simulink model "model_p2"  (R2020b)
settings: Solver=VariableStepAuto  StartTime=0.0  StopTime=10  RelTol=1e-3
model workspace (MAT data in the model file):
  K1 = Simulink.Parameter
  K1.Value = 80000
  K1.DataType = 'auto'
  K1.Dimensions = [1 1]
  K2 = Simulink.Parameter
  K2.Value = 500000
  K2.DataType = 'auto'
  K2.Dimensions = [1 1]
  M1 = Simulink.Parameter
  M1.Value = 2500
  M1.DataType = 'auto'
  M1.Dimensions = [1 1]
  M2 = Simulink.Parameter
  M2.Value = 320
  M2.DataType = 'auto'
  M2.Dimensions = [1 1]
  b = Simulink.Parameter
  b.Value = 350
  b.DataType = 'auto'
  b.Dimensions = [1 1]
settings Model: OrderedModelArguments=off  Creator=ADMIN  LastModifiedBy=ADMIN
settings DataIOCC: ExternalInput=[t, stin]  LoadExternalInput=on  SaveFormat=Array

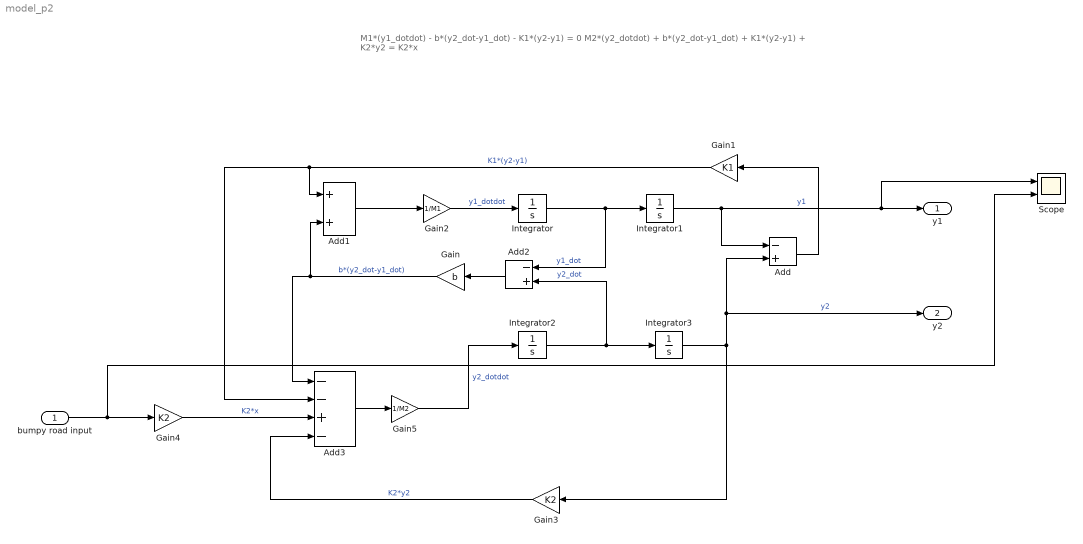
== system model_p2 ==
  note: M1*(y1_dotdot) - b*(y2_dot-y1_dot) - K1*(y2-y1) = 0
      |
      | M2*(y2_dotdot) + b*(y2_dot-y1_dot) + K1*(y2-y1) + K2*y2 = K2*x
  bumpy road input : Inport
  Add : Sum  Inputs=-+
  Add1 : Sum
  Add2 : Sum  Inputs=-+
  Add3 : Sum  Inputs=--+-
  Gain : Gain  Gain=b
  Gain1 : Gain  Gain=K1
  Gain2 : Gain  Gain=1/M1
  Gain3 : Gain  Gain=K2
  Gain4 : Gain  Gain=K2
  Gain5 : Gain  Gain=1/M2
  Integrator{,1..3} (4 alike) : Integrator
  Scope : Scope  NumInputPorts=2
  "y1 " : Outport
  y2 : Outport  Port=2
  wires:
  Gain2/1 -> Integrator/1  "y1_dotdot"
  Integrator/1 -> Add2/1, Integrator1/1  "y1_dot"
  Integrator1/1 -> Add/1, Scope/1, "y1 "/1  "y1"
  Integrator2/1 -> Add2/2, Integrator3/1  "y2_dot"
  Gain5/1 -> Integrator2/1  "y2_dotdot"
  Integrator3/1 -> Gain3/1, Add/2, y2/1  "y2"
  Add/1 -> Gain1/1
  Gain1/1 -> Add3/2, Add1/1  "K1*(y2-y1)"
  Add2/1 -> Gain/1
  Gain/1 -> Add3/1, Add1/2  "b*(y2_dot-y1_dot)"
  Add1/1 -> Gain2/1
  Gain3/1 -> Add3/4  "K2*y2"
  Add3/1 -> Gain5/1
  Gain4/1 -> Add3/3  "K2*x"
  bumpy road input/1 -> Scope/2, Gain4/1
